simulink model "refuel_model"  (R2021b)
settings: Solver=ode15s  StartTime=0.0  StopTime=tsim  MinStep=min_step  RelTol=1e-3  EnableMultiTasking=on
InitFcn:
  | min_step=1e-12;
  | warning 'off';
values from neighbouring files (symbols this model uses):
  area_valve = (pi*dpipe^2/4)    (= 4.90166993776e-05)    [script_compressor.m]    (also in script_refuel.m)
  ki = 0.01/1e3    (= 1e-05)    [script_refuel.m]
  ki_cool = 1e4    (= 10000)    [script_refuel.m]
  Kmin = 0.05    [script_H2_assumption.m]    (also in script_refuel.m = 0.00125)
  kp = 0.01    [script_refuel.m]
  kp_cool = 1e4    (= 10000)    [script_refuel.m]
  Kv1 = 1    [script_H2_assumption.m]    (also in script_compressor.m = 0.025; script_refuel.m = 0.025)
  Kv2 = Kv1    (= 1)    [script_H2_assumption.m]    (also in script_refuel.m = 0.025)
  ph2_rate = 100/60    (= 1.66666666667)    [script_compressor.m]    (also in script_refuel.m)
  R_h2 = 4.12    [script_H2_assumption.m]    (also in script_compressor.m; script_init_pressures.m; script_pipe_dim.m; script_refuel.m)
  tc = 1000    [script_H2_assumption.m]    (also in script_refuel.m)
  tsim = 2000    [script_H2_assumption.m]    (also in script_compressor.m; script_init_pressures.m = 10; script_pipe_dim.m = 30; script_refuel.m)
  vch_o = 0.125    [script_compressor.m]    (also in script_init_pressures.m; script_pipe_dim.m; script_refuel.m)
libraries: fl_lib x36, nesl_utility x7, slpidlib x2, simulink x1
(part 4 of 4)

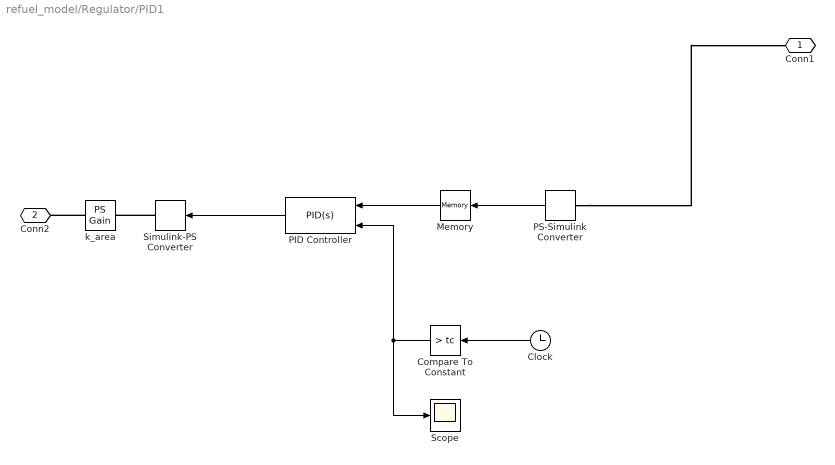
== system refuel_model/Regulator/PID1 ==
  Clock : Clock
  Compare To Constant : simulink/Logic and Bit Operations/Compare To Constant  relop=>  const=tc  OutDataTypeStr=boolean
  Memory : Memory
  PID Controller : slpidlib/PID Controller  Controller=PID  Form=Parallel  TimeDomain=Continuous-time  UseExternalTs=off  SampleTime=-1  IntegratorMethod=Forward Euler  FilterMethod=Forward Euler  ControllerParametersSource=internal  P=kp  I=ki  D=0  UseFilter=on  N=100  TunerSelectOption=Transfer Function Based (PID Tuner App)  InitialConditionSource=internal  InitialConditionForIntegrator=0  InitialConditionForFilter=0  DifferentiatorICPrevScaledInput=0  ExternalReset=either  TrackingMode=off  Kt=1  LimitOutput=on  SatLimitsSource=internal  UpperSaturationLimit=1  LowerSaturationLimit=0  LinearizeAsGain=on  AntiWindupMode=back-calculation  Kb=1e5  POutMin=[]  POutMax=[]  IOutMin=[]  IOutMax=[]  DOutMin=[]  DOutMax=[]  NOutMin=[]  NOutMax=[]  SumOutMin=[]  SumOutMax=[]  SaturationOutMin=[]  SaturationOutMax=[]  PParamMin=[]  PParamMax=[]  IParamMin=[]  IParamMax=[]  DParamMin=[]  DParamMax=[]  NParamMin=[]  NParamMax=[]  KbParamMin=[]  KbParamMax=[]  KtParamMin=[]  KtParamMax=[]  KbOutMin=[]  KbOutMax=[]  KtOutMin=[]  KtOutMax=[]  IntegratorOutMin=[]  IntegratorOutMax=[]  FilterOutMin=[]  FilterOutMax=[]  SumI1OutMin=[]  SumI1OutMax=[]  SumI2OutMin=[]  SumI2OutMax=[]  SumI3OutMin=[]  SumI3OutMax=[]  SumI4OutMin=[]  SumI4OutMax=[]  SumDOutMin=[]  SumDOutMax=[]  DifferentiatorOutMin=[]  DifferentiatorOutMax=[]  FilterDiffOutCoefMin=[]  FilterDiffOutCoefMax=[]  ReciprocalOutMin=[]  ReciprocalOutMax=[]  SumDenOutMin=[]  SumDenOutMax=[]  SumNumOutMin=[]  SumNumOutMax=[]  DivideOutMin=[]  DivideOutMax=[]  UdiffTsProdOutMin=[]  UdiffTsProdOutMax=[]  NTsProdOutMin=[]  NTsProdOutMax=[]  UintegralTsProdOutMin=[]  UintegralTsProdOutMax=[]  UngainTsProdOutMin=[]  UngainTsProdOutMax=[]  IntegratorContinuousStateAttributes=''  IntegratorStateMustResolveToSignalObject=off  IntegratorRTWStateStorageClass=Auto  FilterContinuousStateAttributes=''  FilterStateMustResolveToSignalObject=off  FilterRTWStateStorageClass=Auto  ParallelPVariant=InternalParameters  IdealPVariant=Disabled  IVariant=InternalParameters  DVariant=InternalParameters  IntegratorVariant=Continuous  SatVariant=Enabled  AWVariant=BackCalculation  PCopyVariant=Disabled  TRVariant=Disabled  FdbkBlocksVariant=Forward  IdealPFdbkVariant=Disabled  SatFdbkVariant=Disabled  DerivativeFilterVariant=ContFilter  NVariant=InternalParameters  NCopyVariant=Disabled  FilterICVariant=InternalICsFilter  IntegratorICVariant=InternalICs  ExternalResetVariant=ExternalReset  TRSumVariant=Passthrough  SumFdbkVariant=Disabled  SumVariant=Sum_PID  TsampFilterVariant=InternalTs  TsampNgainVariant=Passthrough  TsampIntegralVariant=Passthrough  ExternalSaturationOutDataTypeStr=Inherit: Same as second input
  PS-Simulink Converter : nesl_utility/PS-Simulink Converter  PhysicalDomain=network_engine_domain  SubClassName=ps_output  LeftPortType=input  RightPortType=output  PseudoPeriodic=off  Frequencies=[]  Unit=bar  AffineConversion=off
      settings: SourceProductBaseCode=PW,SS
  Scope : Scope
  Simulink-PS Converter : nesl_utility/Simulink-PS Converter  PhysicalDomain=network_engine_domain  SubClassName=ps_input  LeftPortType=input  RightPortType=output  PseudoPeriodic=off  Frequencies=[]  NoiseDistribution=none  NoiseParameters=[]  Unit=1  AffineConversion=off  FilteringAndDerivatives=filter  SimscapeFilterOrder=1  InputFilterTimeConstant=0.1  UdotUserProvided=1
      settings: SourceProductBaseCode=PW,SS
  k_area : fl_lib/Physical Signals/Functions/PS Gain  gain=area_valve
  Conn1 : PMIOPort  Side=Right
  Conn2 : PMIOPort  Port=2  Side=Left
  wires:
  PID Controller/1 -> Simulink-PS Converter/1
  PS-Simulink Converter/1 -> Memory/1
  Clock/1 -> Compare To Constant/1
  Compare To Constant/1 -> PID Controller/2, Scope/1
  Memory/1 -> PID Controller/1
  connections:
  PS-Simulink Converter/LConn1 -- Conn1/RConn1
  k_area/RConn1 -- Conn2/RConn1
  Simulink-PS Converter/RConn1 -- k_area/LConn1

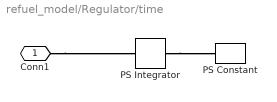
== system refuel_model/Regulator/time ==
  PS Constant : fl_lib/Physical Signals/Sources/PS Constant  constant=1
  PS Integrator : fl_lib/Physical Signals/Linear Operators/PS Integrator  reset_method=foundation.enum.IntegratorResetSpec.None  initial_condition_spec=foundation.enum.IntegratorICSpec.Internal  x0=0 s
      settings: SourceProductBaseCode=SS
  Conn1 : PMIOPort  Side=Left
  connections:
  Conn1/RConn1 -- PS Integrator/RConn1
  PS Integrator/LConn1 -- PS Constant/RConn1
